simulink model "Simulation"  (R2022b)
settings: Solver=FixedStepAuto  StartTime=0.0  StopTime=200  FixedStep=0.01  RelTol=1e-3
values from neighbouring files (symbols this model uses):
  A = [0 1;-k/m -c/m]    [Main_Euler.m]    (also in main.m = zeros(n,n))
  B = [1/m]    [Main_Euler.m]    (also in main.m = zeros(n,m))
  g = 9.81    [main.m]
  K = place(A,B,[-10 -2 -10 -3 -100 -1])    [main.m]
  mass = 1    [main.m]
  x = y*0    [animation.m]    (also in mian.mat = [10 10.009451667 10.0178133394 10.0250950312 10.031306764 10)
settings Model: Creator=baj1377  LastModifiedBy=baj1377

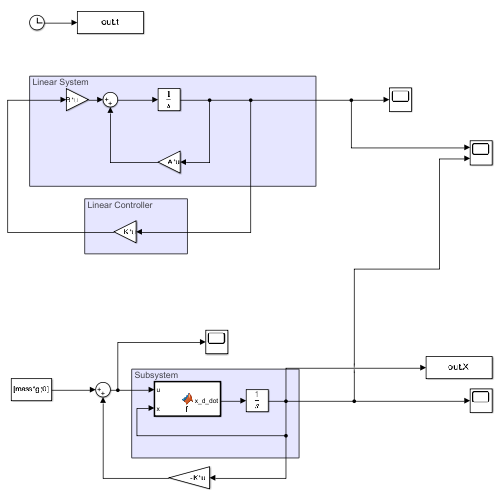
[thumbnail: Simulink's stored preview of the top-level diagram]
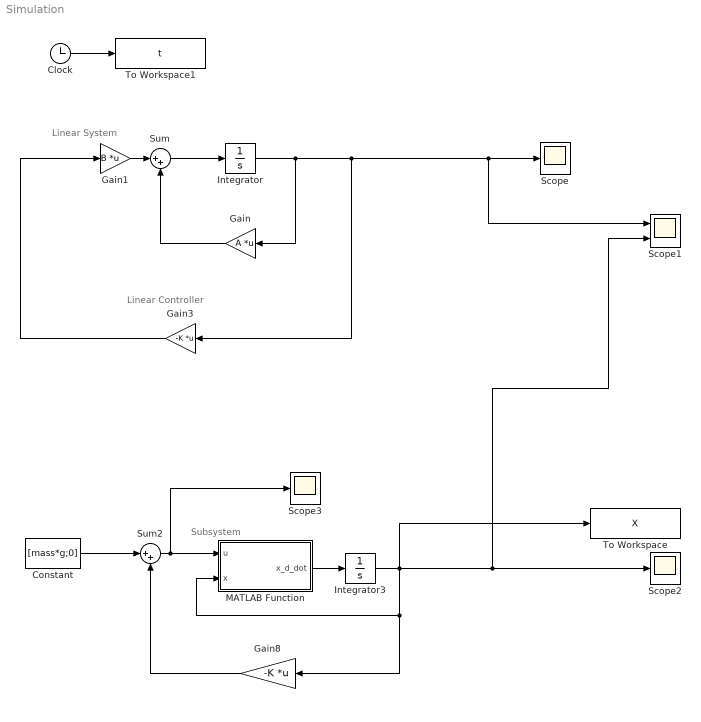
== system Simulation ==
  note: Subsystem
  note: Linear Controller
  note: Linear System
  Clock : Clock
  Constant : Constant  Value=[mass*g;0]
  Gain : Gain  Gain=A  Multiplication=Matrix(K*u)
  Gain1 : Gain  Gain=B  Multiplication=Matrix(K*u)
  Gain3 : Gain  Gain=-K  Multiplication=Matrix(K*u)
  Gain8 : Gain  Gain=-K  Multiplication=Matrix(K*u)
  Integrator : Integrator  InitialCondition=x(:,1)
  Integrator3 : Integrator  InitialCondition=x(:,1)
  MATLAB Function : MATLAB Function  TreatAsAtomicUnit=on
  Scope : Scope
  Scope1 : Scope  NumInputPorts=2
  Scope2 : Scope
  Scope3 : Scope
  Sum : Sum  Inputs=|++
  Sum2 : Sum  Inputs=|++
  To Workspace : ToWorkspace  VariableName=X  SampleTime=0.01
  To Workspace1 : ToWorkspace  VariableName=t  SampleTime=0.01
      settings: Save2DSignal=2-D array (concatenate along first dimension)
  wires:
  Integrator/1 -> Scope1/1, Scope/1, Gain3/1, Gain/1
  Sum/1 -> Integrator/1
  Gain1/1 -> Sum/1
  Gain/1 -> Sum/2
  Constant/1 -> Sum2/1
  Integrator3/1 -> Scope1/2, Scope2/1, To Workspace/1, Gain8/1, MATLAB Function/2(x)
  Gain8/1 -> Sum2/2
  Clock/1 -> To Workspace1/1
  Gain3/1 -> Gain1/1
  Sum2/1 -> Scope3/1, MATLAB Function/1(u)
  MATLAB Function/1(x_d_dot) -> Integrator3/1

== matlab function Simulation/MATLAB Function ==
  data: u input; x input; x_d_dot output
function x_d_dot = f(u,x)
mass = 1; I = 1e-4; l =0.1;g=9.81;

x_d_dot = [x(2);-u(1)/mass*sin(x(5));x(4);u(1)/mass*cos(x(5))-g;x(6);l/(2*I)*u(2)];
